simulink model "CLIK_TRNS"  (R2023a)
settings: Solver=ode1  StartTime=0.0  StopTime=25  FixedStep=Ts  RelTol=1e-3
values from neighbouring files (symbols this model uses):
  Ts = 0.001    [TRAJ.m]
undefined symbols (not defined in the file or in its folder): DiscIntNeverNeededParam
settings Model: Creator=39388  LastModifiedBy=39388

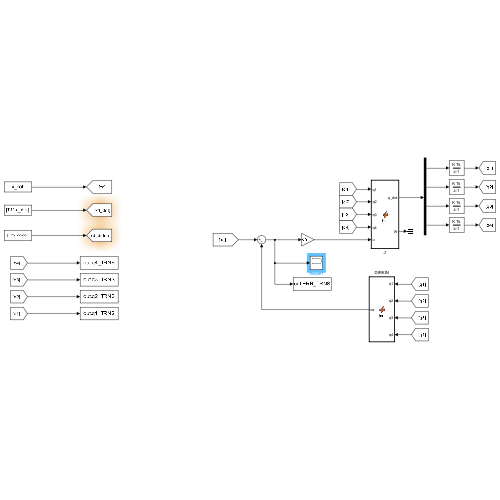
[thumbnail: Simulink's stored preview of the top-level diagram]
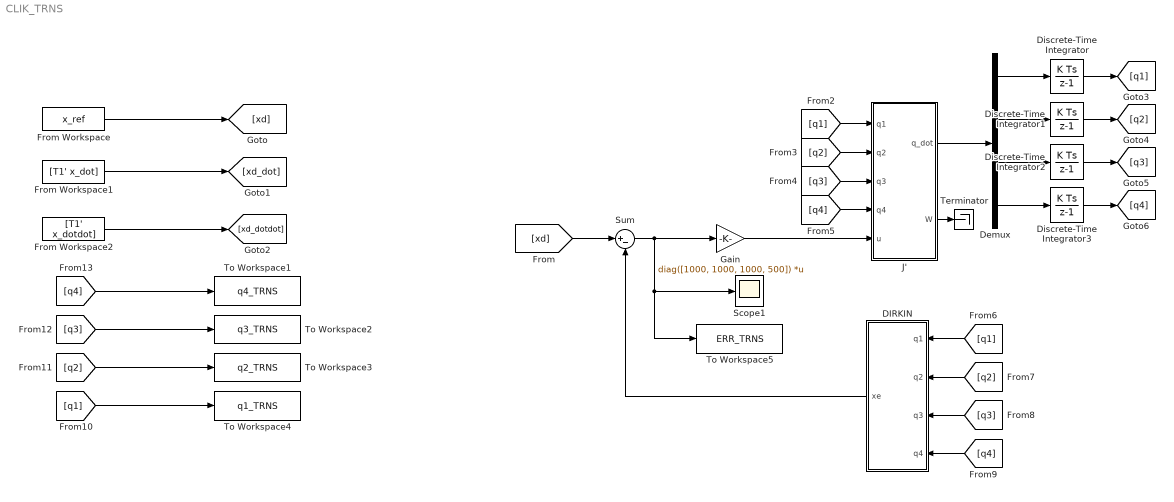
== system CLIK_TRNS ==
  DIRKIN : MATLAB Function  TreatAsAtomicUnit=on
  Demux : Demux
  Discrete-Time Integrator : DiscreteIntegrator  SampleTime=Ts  ICPrevOutput=DiscIntNeverNeededParam  ICPrevScaledInput=DiscIntNeverNeededParam
  Discrete-Time Integrator1 : DiscreteIntegrator  InitialCondition=pi/2  SampleTime=Ts  ICPrevOutput=DiscIntNeverNeededParam  ICPrevScaledInput=DiscIntNeverNeededParam
  Discrete-Time Integrator2 : DiscreteIntegrator  InitialCondition=-0.25  SampleTime=Ts  ICPrevOutput=DiscIntNeverNeededParam  ICPrevScaledInput=DiscIntNeverNeededParam
  Discrete-Time Integrator3 : DiscreteIntegrator  InitialCondition=-pi  SampleTime=Ts  ICPrevOutput=DiscIntNeverNeededParam  ICPrevScaledInput=DiscIntNeverNeededParam
  From Workspace : FromWorkspace  VariableName=x_ref
  From Workspace1 : FromWorkspace  VariableName=[T1' x_dot]
  From Workspace2 : FromWorkspace  VariableName=[T1' x_dotdot]
  Gain : Gain  Gain=diag([1000, 1000, 1000, 500])  Multiplication=Matrix(K*u)
  J' : MATLAB Function  TreatAsAtomicUnit=on
  Scope1 : Scope
  Sum : Sum  Inputs=|+-
  Terminator : Terminator
  To Workspace1 : ToWorkspace  VariableName=q4_TRNS  SaveFormat=Structure With Time  SampleTime=-1
  To Workspace2 : ToWorkspace  VariableName=q3_TRNS  SaveFormat=Structure With Time  SampleTime=-1
  To Workspace3 : ToWorkspace  VariableName=q2_TRNS  SaveFormat=Structure With Time  SampleTime=-1
  To Workspace4 : ToWorkspace  VariableName=q1_TRNS  SaveFormat=Structure With Time  SampleTime=-1
  To Workspace5 : ToWorkspace  VariableName=ERR_TRNS  SaveFormat=Structure With Time  SampleTime=-1
  wires:
  From Workspace1/1 -> [xd_dot]
  From Workspace2/1 -> [xd_dotdot]
  [xd] -> Sum/1
  Sum/1 -> To Workspace5/1, Scope1/1, Gain/1
  Gain/1 -> J'/5(u)
  DIRKIN/1(xe) -> Sum/2
  From Workspace/1 -> [xd]
  J'/1(q_dot) -> Demux/1
  Demux/1 -> Discrete-Time Integrator/1
  Demux/2 -> Discrete-Time Integrator1/1
  Demux/3 -> Discrete-Time Integrator2/1
  Demux/4 -> Discrete-Time Integrator3/1
  Discrete-Time Integrator/1 -> [q1]
  Discrete-Time Integrator1/1 -> [q2]
  Discrete-Time Integrator2/1 -> [q3]
  Discrete-Time Integrator3/1 -> [q4]
  [q1] -> J'/1(q1)
  [q2] -> J'/2(q2)
  [q3] -> J'/3(q3)
  [q4] -> J'/4(q4)
  [q1] -> DIRKIN/1(q1)
  [q2] -> DIRKIN/2(q2)
  [q3] -> DIRKIN/3(q3)
  [q4] -> DIRKIN/4(q4)
  [q4] -> To Workspace1/1
  [q3] -> To Workspace2/1
  [q2] -> To Workspace3/1
  [q1] -> To Workspace4/1
  J'/2(W) -> Terminator/1

== matlab function CLIK_TRNS/DIRKIN ==
  data: q1 input; xe output; q2 input; q3 input; q4 input
function xe = fcn(q1,q2,q3,q4)

xe=[0.5*cos(q1)+0.5*cos(q1+q2);
    0.5*sin(q1)+0.5*sin(q1+q2);
    1+q3;
    q1+q2+q4];

== matlab function CLIK_TRNS/J' ==
  data: q1 input; q2 input; q3 input; q4 input; u input; q_dot output; W output
function  [q_dot,W] = fcn(q1,q2,q3,q4,u)

    J=[-0.5*sin(q1-0.5*sin(q1+q2)) -0.5*sin(q1+q2) 0 0;
        0.5*cos(q1-0.5*cos(q1+q2))  0.5*cos(q1+q2) 0 0;
        0                               0                 1 0;
        1                               1                 0 1];

     q_dot=J'*u;
     W=0.5^2*0.5^2*(sin(q2))^2;
